simulink model "ex4"  (R2014a)
settings: Solver=ode45  StartTime=0.0  StopTime=3  RelTol=1e-3
settings Model: Creator=liang  LastModifiedBy=liang

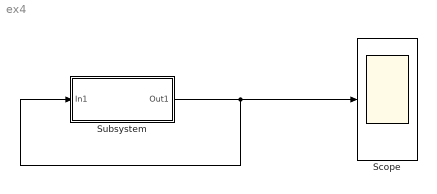
== system ex4 ==
  Scope : Scope
      settings: MaxDataPoints=50000
  Subsystem : Subsystem
  wires:
  Subsystem/1(Out1) -> Scope/1, Subsystem/1(In1)

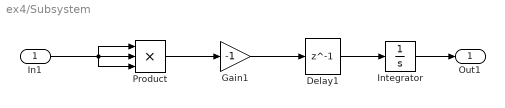
== system ex4/Subsystem ==
  In1 : Inport
  Delay1 : Delay  DelayLength=1  SampleTime=0.001
  Gain1 : Gain  Gain=-1
  Integrator : Integrator  InitialCondition=200
  Product : Product  Inputs=3
  Out1 : Outport
  wires:
  Integrator/1 -> Out1/1
  Delay1/1 -> Integrator/1
  Gain1/1 -> Delay1/1
  In1/1 -> Product/3, Product/2, Product/1
  Product/1 -> Gain1/1
